simulink model "B34CostaTest"  (R2023a)
settings: Solver=VariableStepAuto  StartTime=0.0  StopTime=100  RelTol=1E-4  AbsTol=1E-4
values from neighbouring files (symbols this model uses):
  AinfK_h_B34 = -25    [B34.m]
  AinfK_p_B34 = 1.0    (= 1)    [B34.m]
  AinfK_s_B34 = 9.0    (= 9)    [B34.m]
  AinfKA_h_B34 = -60    [B34.m]    (also in CtrlParaSNSTuning.m)
  AinfKA_p_B34 = 1.0    (= 1)    [B34.m]    (also in CtrlParaSNSTuning.m)
  AinfKA_s_B34 = 1.0    (= 1)    [B34.m]    (also in CtrlParaSNSTuning.m)
  AinfNa_h_B34 = -39    [B34.m]
  AinfNa_p_B34 = 1.0    (= 1)    [B34.m]
  AinfNa_s_B34 = 5.0    (= 5)    [B34.m]
  AK_B34_0 = 0.4    [B34.m]
  AKA_B34_0 = 0.4    [B34.m]    (also in CtrlParaSNSTuning.m; InitPara.m)
  ANa_B34_0 = 0.4    [B34.m]
  BinfKA_h_B34 = -55.0    (= -55)    [B34.m]    (also in CtrlParaSNSTuning.m)
  BinfKA_p_B34 = 2.0    (= 2)    [B34.m]    (also in CtrlParaSNSTuning.m)
  BinfKA_s_B34 = 1.0    (= 1)    [B34.m]    (also in CtrlParaSNSTuning.m)
  BinfNa_h_B34 = -45.0    (= -45)    [B34.m]
  BinfNa_p_B34 = 1.0    (= 1)    [B34.m]
  BinfNa_s_B34 = 5.0    (= 5)    [B34.m]
  BKA_B34_0 = 0.4    [B34.m]    (also in CtrlParaSNSTuning.m; InitPara.m)
  BNa_B34_0 = 0.4    [B34.m]
  Cm_B34 = 0.01    [B34.m]    (also in CtrlParaSNSTuning.m)
  EK_B34 = -70    [B34.m]
  EKA_B34 = -60    [B34.m]    (also in CtrlParaSNSTuning.m)
  EL_B34 = -60    [B34.m]    (also in CtrlParaSNSTuning.m)
  ENa_B34 = 30    [B34.m]
  gK_B34 = 13    [B34.m]
  gKA_B34 = 1.25    [B34.m]    (also in CtrlParaSNSTuning.m)
  gL_B34 = 0.1    [B34.m]    (also in CtrlParaSNSTuning.m)
  gNa_B34 = 25    [B34.m]
  pK_B34 = 4    [B34.m]
  pKA_B34 = 2    [B34.m]    (also in CtrlParaSNSTuning.m)
  pNa_B34 = 3    [B34.m]
  RK_B34 = 0    [B34.m]
  RKA_B34 = 0    [B34.m]    (also in CtrlParaSNSTuning.m)
  RL_B34 = 0    [B34.m]    (also in CtrlParaSNSTuning.m)
  RNa_B34 = 0    [B34.m]
  tAK_h_B34 = -10.0    (= -10)    [B34.m]
  tAK_p_B34 = 1.0    (= 1)    [B34.m]
  tAK_s_B34 = 10.0    (= 10)    [B34.m]
  tAK_tmax_B34 = 0.04    [B34.m]
  tAK_tmin_B34 = 0.004    [B34.m]
  tAKA_h_B34 = -56    [B34.m]    (also in CtrlParaSNSTuning.m)
  tAKA_p_B34 = 2.0    (= 2)    [B34.m]    (also in CtrlParaSNSTuning.m)
  tAKA_s_B34 = 1.0    (= 1)    [B34.m]    (also in CtrlParaSNSTuning.m)
  tAKA_tmax_B34 = 0.2    [B34.m]    (also in CtrlParaSNSTuning.m)
  tAKA_tmin_B34 = 0.02    [B34.m]    (also in CtrlParaSNSTuning.m)
  tANa_h_B34 = -45    [B34.m]
  tANa_p_B34 = 1.0    (= 1)    [B34.m]
  tANa_s_B34 = 4.0    (= 4)    [B34.m]
  tANa_tmax_B34 = 0.006    [B34.m]
  tANa_tmin_B34 = 0.001    [B34.m]
  tBKA_tmax_B34 = 0.5    [B34.m]    (also in CtrlParaSNSTuning.m)
  tBNa_h_B34 = -40    [B34.m]
  tBNa_p_B34 = 1.0    (= 1)    [B34.m]
  tBNa_s_B34 = 10.0    (= 10)    [B34.m]
  tBNa_tmax_B34 = 0.02    [B34.m]
  tBNa_tmin_B34 = 0.005    [B34.m]
  V_B34_0 = -60    [B34.m]    (also in CtrlParaSNSTuning.m; InitPara.m)
undefined symbols (not defined in the file or in its folder): Iapp
settings Model: SimulationMode=accelerator  Creator=liyan  LastModifiedBy=Yanjun
settings ModelReferenceCC: EnableRefExpFcnMdlSchedulingChecks=on

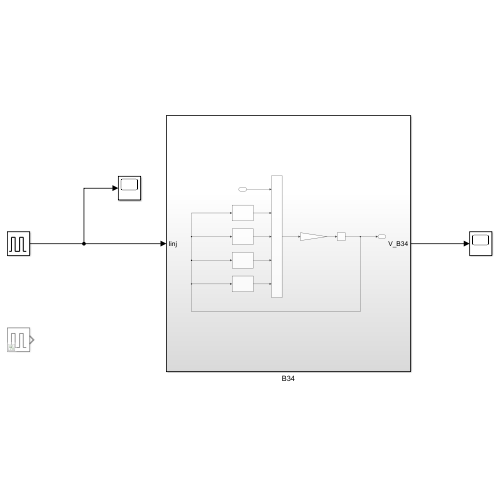
[thumbnail: Simulink's stored preview of the top-level diagram]
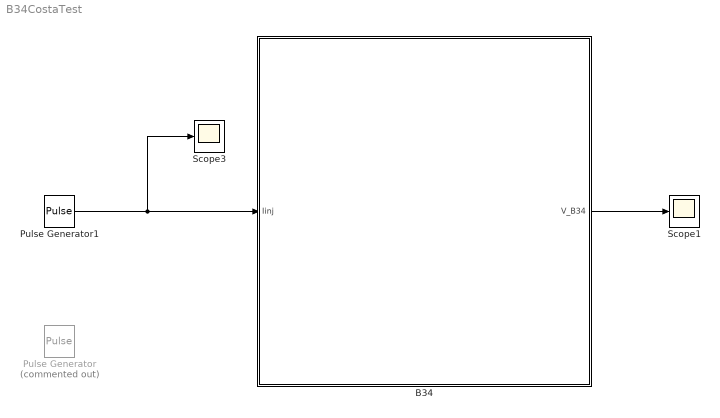
== system B34CostaTest ==
  B34 : Subsystem
  Pulse Generator : DiscretePulseGenerator  Commented=on  PulseType=Time based  Amplitude=Iapp  Period=30  PulseWidth=10/30*100  PhaseDelay=10
  Pulse Generator1 : DiscretePulseGenerator  PulseType=Time based  Amplitude=Iapp  Period=100  PulseWidth=10/100*100  PhaseDelay=35
  Scope1 : Scope
  Scope3 : Scope
  wires:
  Pulse Generator1/1 -> Scope3/1, B34/1(Iinj)
  B34/1(V_B34) -> Scope1/1

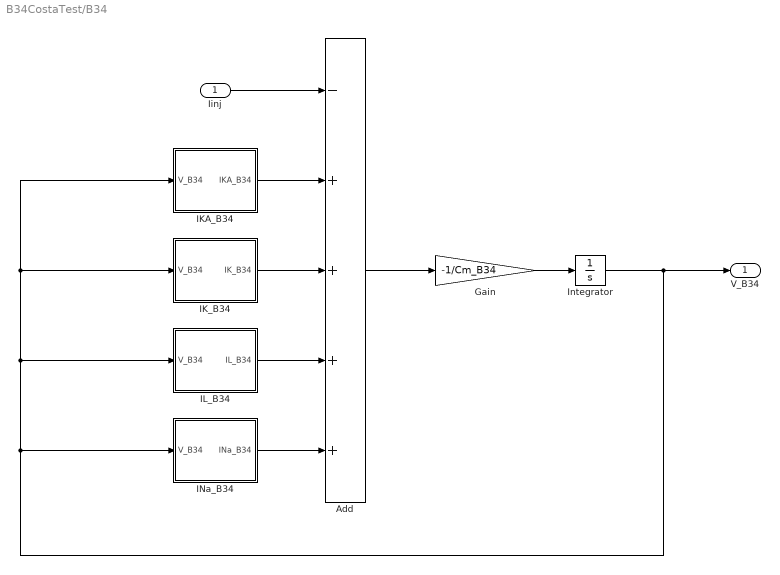
== system B34CostaTest/B34 ==
  Iinj : Inport
  Add : Sum  Inputs=-++++
  Gain : Gain  Gain=-1/Cm_B34
  IKA_B34 : Subsystem
  IK_B34 : Subsystem
  IL_B34 : Subsystem
  INa_B34 : Subsystem
  Integrator : Integrator  InitialCondition=V_B34_0
  V_B34 : Outport
  wires:
  Gain/1 -> Integrator/1
  Add/1 -> Gain/1
  Integrator/1 -> INa_B34/1(V_B34), IK_B34/1(V_B34), IKA_B34/1(V_B34), IL_B34/1(V_B34), V_B34/1
  IKA_B34/1(IKA_B34) -> Add/2
  IK_B34/1(IK_B34) -> Add/3
  IL_B34/1(IL_B34) -> Add/4
  INa_B34/1(INa_B34) -> Add/5
  Iinj/1 -> Add/1

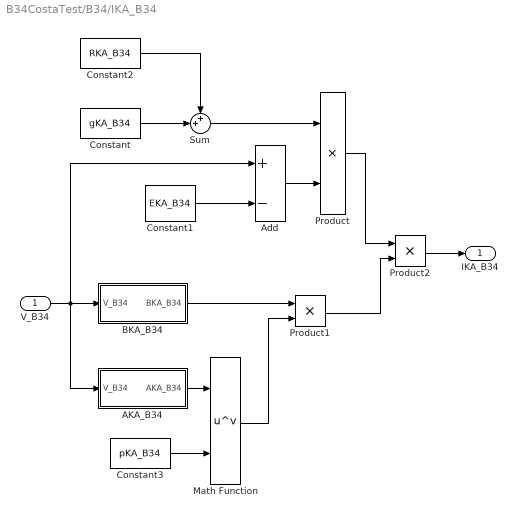
== system B34CostaTest/B34/IKA_B34 ==
  V_B34 : Inport
  AKA_B34 : Subsystem
  Add : Sum  Inputs=+-
  BKA_B34 : Subsystem
  Constant : Constant  Value=gKA_B34
  Constant1 : Constant  Value=EKA_B34
  Constant2 : Constant  Value=RKA_B34
  Constant3 : Constant  Value=pKA_B34
  Math Function : Math  Operator=pow
  Product : Product
  Product1 : Product
  Product2 : Product
  Sum : Sum  Inputs=++|
  IKA_B34 : Outport
  wires:
  Add/1 -> Product/2
  Constant1/1 -> Add/2
  V_B34/1 -> AKA_B34/1(V_B34), BKA_B34/1(V_B34), Add/1
  Product/1 -> Product2/1
  Product1/1 -> Product2/2
  Product2/1 -> IKA_B34/1
  Constant/1 -> Sum/2
  Sum/1 -> Product/1
  Constant2/1 -> Sum/1
  AKA_B34/1(AKA_B34) -> Math Function/1
  Constant3/1 -> Math Function/2
  BKA_B34/1(BKA_B34) -> Product1/1
  Math Function/1 -> Product1/2

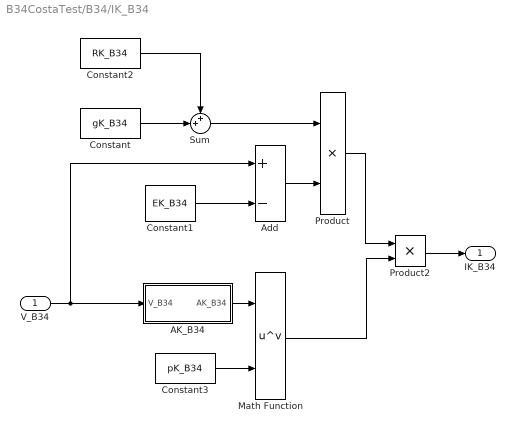
== system B34CostaTest/B34/IK_B34 ==
  V_B34 : Inport
  AK_B34 : Subsystem
  Add : Sum  Inputs=+-
  Constant : Constant  Value=gK_B34
  Constant1 : Constant  Value=EK_B34
  Constant2 : Constant  Value=RK_B34
  Constant3 : Constant  Value=pK_B34
  Math Function : Math  Operator=pow
  Product : Product
  Product2 : Product
  Sum : Sum  Inputs=++|
  IK_B34 : Outport
  wires:
  Add/1 -> Product/2
  Constant1/1 -> Add/2
  V_B34/1 -> AK_B34/1(V_B34), Add/1
  Product/1 -> Product2/1
  Math Function/1 -> Product2/2
  Product2/1 -> IK_B34/1
  Constant/1 -> Sum/2
  Sum/1 -> Product/1
  Constant2/1 -> Sum/1
  AK_B34/1(AK_B34) -> Math Function/1
  Constant3/1 -> Math Function/2

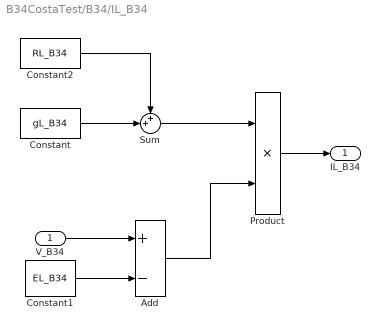
== system B34CostaTest/B34/IL_B34 ==
  V_B34 : Inport
  Add : Sum  Inputs=+-
  Constant : Constant  Value=gL_B34
  Constant1 : Constant  Value=EL_B34
  Constant2 : Constant  Value=RL_B34
  Product : Product
  Sum : Sum  Inputs=++|
  IL_B34 : Outport
  wires:
  Constant1/1 -> Add/2
  V_B34/1 -> Add/1
  Constant2/1 -> Sum/1
  Sum/1 -> Product/1
  Constant/1 -> Sum/2
  Add/1 -> Product/2
  Product/1 -> IL_B34/1

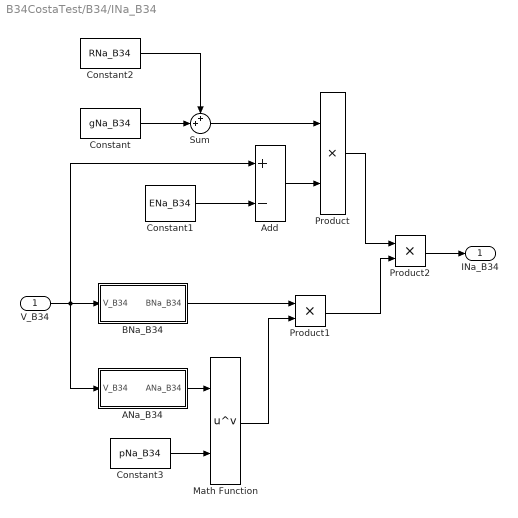
== system B34CostaTest/B34/INa_B34 ==
  V_B34 : Inport
  ANa_B34 : Subsystem
  Add : Sum  Inputs=+-
  BNa_B34 : Subsystem
  Constant : Constant  Value=gNa_B34
  Constant1 : Constant  Value=ENa_B34
  Constant2 : Constant  Value=RNa_B34
  Constant3 : Constant  Value=pNa_B34
  Math Function : Math  Operator=pow
  Product : Product
  Product1 : Product
  Product2 : Product
  Sum : Sum  Inputs=++|
  INa_B34 : Outport
  wires:
  Add/1 -> Product/2
  Constant1/1 -> Add/2
  V_B34/1 -> ANa_B34/1(V_B34), BNa_B34/1(V_B34), Add/1
  Product/1 -> Product2/1
  Product1/1 -> Product2/2
  Product2/1 -> INa_B34/1
  Constant/1 -> Sum/2
  Sum/1 -> Product/1
  Constant2/1 -> Sum/1
  ANa_B34/1(ANa_B34) -> Math Function/1
  Constant3/1 -> Math Function/2
  BNa_B34/1(BNa_B34) -> Product1/1
  Math Function/1 -> Product1/2

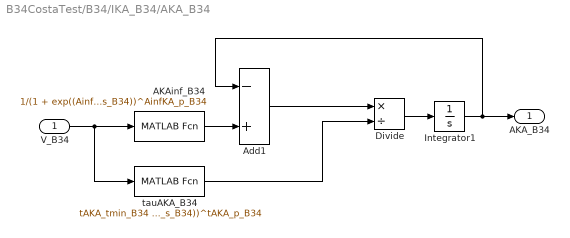
== system B34CostaTest/B34/IKA_B34/AKA_B34 ==
  V_B34 : Inport
  AKAinf_B34 : MATLABFcn  MATLABFcn=1/(1 + exp((AinfKA_h_B34 - u(1))/AinfKA_s_B34))^AinfKA_p_B34
  Add1 : Sum  Inputs=-+
  Divide : Product  Inputs=*/
  Integrator1 : Integrator  InitialCondition=AKA_B34_0
  tauAKA_B34 : MATLABFcn  MATLABFcn=tAKA_tmin_B34 + (tAKA_tmax_B34 - tAKA_tmin_B34)/(1 + exp((u(1) - tAKA_h_B34)/tAKA_s_B34))^tAKA_p_B34
  AKA_B34 : Outport
  wires:
  tauAKA_B34/1 -> Divide/2
  Divide/1 -> Integrator1/1
  V_B34/1 -> tauAKA_B34/1, AKAinf_B34/1
  Integrator1/1 -> Add1/1, AKA_B34/1
  Add1/1 -> Divide/1
  AKAinf_B34/1 -> Add1/2

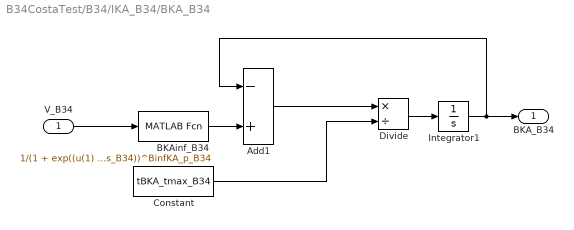
== system B34CostaTest/B34/IKA_B34/BKA_B34 ==
  V_B34 : Inport
  Add1 : Sum  Inputs=-+
  BKAinf_B34 : MATLABFcn  MATLABFcn=1/(1 + exp((u(1) - BinfKA_h_B34)/BinfKA_s_B34))^BinfKA_p_B34
  Constant : Constant  Value=tBKA_tmax_B34
  Divide : Product  Inputs=*/
  Integrator1 : Integrator  InitialCondition=BKA_B34_0
  BKA_B34 : Outport
  wires:
  Constant/1 -> Divide/2
  Divide/1 -> Integrator1/1
  V_B34/1 -> BKAinf_B34/1
  Integrator1/1 -> Add1/1, BKA_B34/1
  Add1/1 -> Divide/1
  BKAinf_B34/1 -> Add1/2

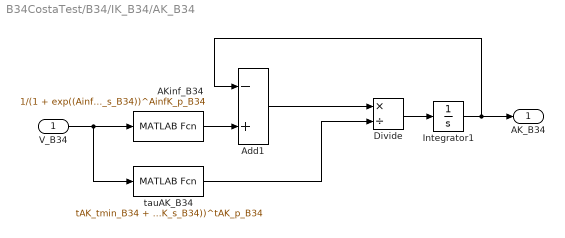
== system B34CostaTest/B34/IK_B34/AK_B34 ==
  V_B34 : Inport
  AKinf_B34 : MATLABFcn  MATLABFcn=1/(1 + exp((AinfK_h_B34 - u(1))/AinfK_s_B34))^AinfK_p_B34
  Add1 : Sum  Inputs=-+
  Divide : Product  Inputs=*/
  Integrator1 : Integrator  InitialCondition=AK_B34_0
  tauAK_B34 : MATLABFcn  MATLABFcn=tAK_tmin_B34 + (tAK_tmax_B34 - tAK_tmin_B34)/(1 + exp((u(1) - tAK_h_B34)/tAK_s_B34))^tAK_p_B34
  AK_B34 : Outport
  wires:
  tauAK_B34/1 -> Divide/2
  Divide/1 -> Integrator1/1
  V_B34/1 -> tauAK_B34/1, AKinf_B34/1
  Integrator1/1 -> Add1/1, AK_B34/1
  Add1/1 -> Divide/1
  AKinf_B34/1 -> Add1/2

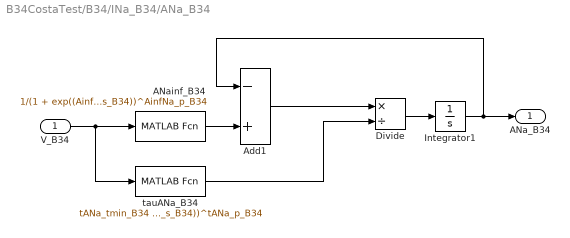
== system B34CostaTest/B34/INa_B34/ANa_B34 ==
  V_B34 : Inport
  ANainf_B34 : MATLABFcn  MATLABFcn=1/(1 + exp((AinfNa_h_B34 - u(1))/AinfNa_s_B34))^AinfNa_p_B34
  Add1 : Sum  Inputs=-+
  Divide : Product  Inputs=*/
  Integrator1 : Integrator  InitialCondition=ANa_B34_0
  tauANa_B34 : MATLABFcn  MATLABFcn=tANa_tmin_B34 + (tANa_tmax_B34 - tANa_tmin_B34)/(1 + exp((u(1) - tANa_h_B34)/tANa_s_B34))^tANa_p_B34
  ANa_B34 : Outport
  wires:
  tauANa_B34/1 -> Divide/2
  Divide/1 -> Integrator1/1
  V_B34/1 -> tauANa_B34/1, ANainf_B34/1
  Integrator1/1 -> Add1/1, ANa_B34/1
  Add1/1 -> Divide/1
  ANainf_B34/1 -> Add1/2

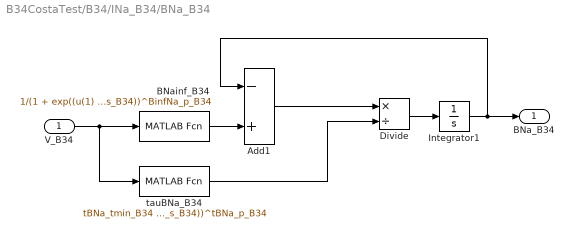
== system B34CostaTest/B34/INa_B34/BNa_B34 ==
  V_B34 : Inport
  Add1 : Sum  Inputs=-+
  BNainf_B34 : MATLABFcn  MATLABFcn=1/(1 + exp((u(1) - BinfNa_h_B34)/BinfNa_s_B34))^BinfNa_p_B34
  Divide : Product  Inputs=*/
  Integrator1 : Integrator  InitialCondition=BNa_B34_0
  tauBNa_B34 : MATLABFcn  MATLABFcn=tBNa_tmin_B34 + (tBNa_tmax_B34 - tBNa_tmin_B34)/(1 + exp((u(1) - tBNa_h_B34)/tBNa_s_B34))^tBNa_p_B34
  BNa_B34 : Outport
  wires:
  tauBNa_B34/1 -> Divide/2
  Divide/1 -> Integrator1/1
  V_B34/1 -> tauBNa_B34/1, BNainf_B34/1
  Integrator1/1 -> Add1/1, BNa_B34/1
  Add1/1 -> Divide/1
  BNainf_B34/1 -> Add1/2
